simulink model "wipers_subsytem"  (R2018a)
settings: Solver=VariableStepAuto  StartTime=0.0  StopTime=inf  RelTol=1e-3
settings Model: DataTypeOverride=Double  MinMaxOverflowLogging=ForceOff  Creator=99003196  LastModifiedBy=99003188
settings DataIOCC: ReturnWorkspaceOutputs=on
settings SFSimCC: SimUseLocalCustomCode=on
settings RTWCC: RTWUseLocalCustomCode=on

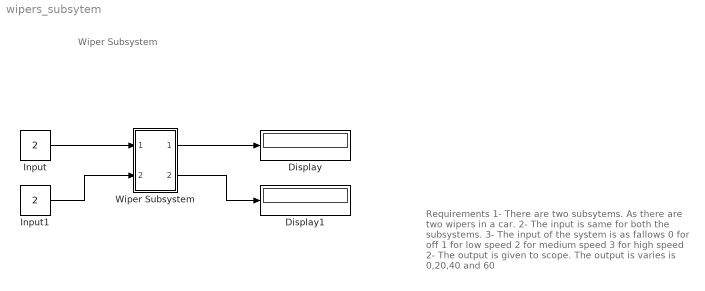
== system wipers_subsytem ==
  note: Wiper Subsystem
  note: Requirements
      | 1- There are two subsytems. As
      | there are two wipers in a car.
      | 2- The input is same for both
      | the subsystems.
      | 3- The input of the system is as fallows
      | 0 for off
      | 1 for low speed
      | 2 for medium speed
      | 3 for high speed
      | 2- The output is given to scope. The output is
      | varies is 0,20,40 and 60
  Display : Display
  Display1 : Display
  Input : Constant  Value=2
  Input1 : Constant  Value=2
  Wiper Subsystem : Subsystem
  wires:
  Input/1 -> Wiper Subsystem/1(In1)
  Wiper Subsystem/1(Out1) -> Display/1
  Input1/1 -> Wiper Subsystem/2(In2)
  Wiper Subsystem/2(Out2) -> Display1/1

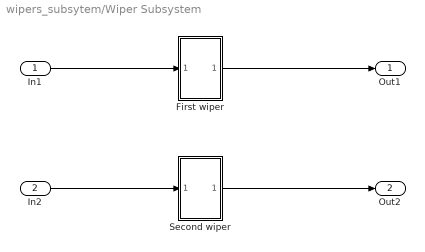
== system wipers_subsytem/Wiper Subsystem ==
  In1 : Inport
  In2 : Inport  Port=2
  First wiper : Subsystem
  Second wiper : Subsystem
  Out1 : Outport
  Out2 : Outport  Port=2
  wires:
  In1/1 -> First wiper/1(In1)
  First wiper/1(Out1) -> Out1/1
  Second wiper/1(Out1) -> Out2/1
  In2/1 -> Second wiper/1(In1)

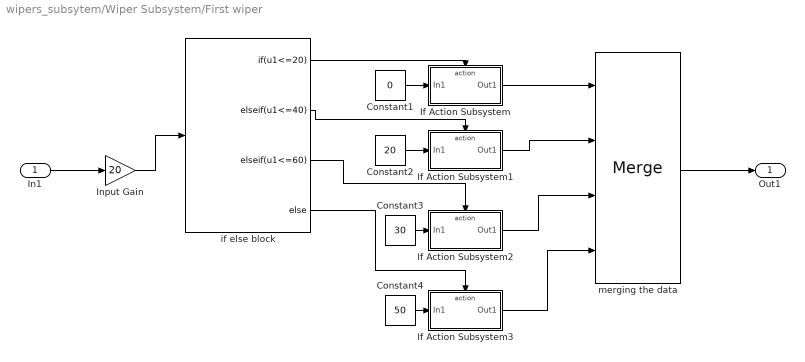
== system wipers_subsytem/Wiper Subsystem/First wiper ==
  In1 : Inport
  Constant1 : Constant  Value=0
  Constant2 : Constant  Value=20
  Constant3 : Constant  Value=30
  Constant4 : Constant  Value=50
  If Action Subsystem : Subsystem  TreatAsAtomicUnit=on
  If Action Subsystem1 : Subsystem  TreatAsAtomicUnit=on
  If Action Subsystem2 : Subsystem  TreatAsAtomicUnit=on
  If Action Subsystem3 : Subsystem  TreatAsAtomicUnit=on
  Input Gain : Gain  Gain=20
  if else block : If  IfExpression=u1<=20  ElseIfExpressions=u1<=40,u1<=60
  "merging the data " : Merge  Inputs=4
  Out1 : Outport
  wires:
  if else block/2 -> If Action Subsystem1/Action
  If Action Subsystem3/1(Out1) -> "merging the data "/4
  if else block/1 -> If Action Subsystem/Action
  if else block/3 -> If Action Subsystem2/Action
  Constant4/1 -> If Action Subsystem3/1(In1)
  If Action Subsystem/1(Out1) -> "merging the data "/1
  Constant3/1 -> If Action Subsystem2/1(In1)
  If Action Subsystem1/1(Out1) -> "merging the data "/2
  Input Gain/1 -> if else block/1
  If Action Subsystem2/1(Out1) -> "merging the data "/3
  "merging the data "/1 -> Out1/1
  In1/1 -> Input Gain/1
  Constant2/1 -> If Action Subsystem1/1(In1)
  Constant1/1 -> If Action Subsystem/1(In1)
  if else block/4 -> If Action Subsystem3/Action

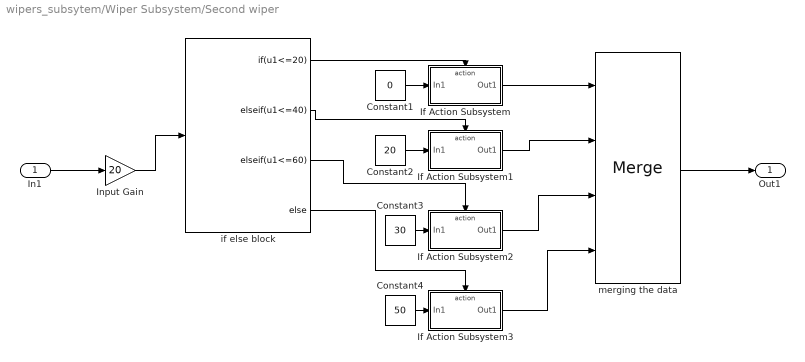
== system wipers_subsytem/Wiper Subsystem/Second wiper ==
  In1 : Inport
  Constant1 : Constant  Value=0
  Constant2 : Constant  Value=20
  Constant3 : Constant  Value=30
  Constant4 : Constant  Value=50
  If Action Subsystem : Subsystem  TreatAsAtomicUnit=on
  If Action Subsystem1 : Subsystem  TreatAsAtomicUnit=on
  If Action Subsystem2 : Subsystem  TreatAsAtomicUnit=on
  If Action Subsystem3 : Subsystem  TreatAsAtomicUnit=on
  Input Gain : Gain  Gain=20
  if else block : If  IfExpression=u1<=20  ElseIfExpressions=u1<=40,u1<=60
  "merging the data " : Merge  Inputs=4
  Out1 : Outport
  wires:
  if else block/2 -> If Action Subsystem1/Action
  If Action Subsystem3/1(Out1) -> "merging the data "/4
  if else block/1 -> If Action Subsystem/Action
  if else block/3 -> If Action Subsystem2/Action
  Constant4/1 -> If Action Subsystem3/1(In1)
  If Action Subsystem/1(Out1) -> "merging the data "/1
  Constant3/1 -> If Action Subsystem2/1(In1)
  If Action Subsystem1/1(Out1) -> "merging the data "/2
  Input Gain/1 -> if else block/1
  If Action Subsystem2/1(Out1) -> "merging the data "/3
  "merging the data "/1 -> Out1/1
  In1/1 -> Input Gain/1
  Constant2/1 -> If Action Subsystem1/1(In1)
  Constant1/1 -> If Action Subsystem/1(In1)
  if else block/4 -> If Action Subsystem3/Action

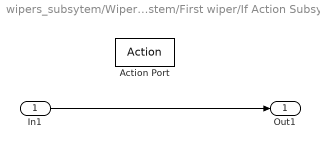
== system wipers_subsytem/Wiper Subsystem/First wiper/If Action Subsystem ==
  In1 : Inport
  Action Port : ActionPort
  Out1 : Outport
  wires:
  In1/1 -> Out1/1

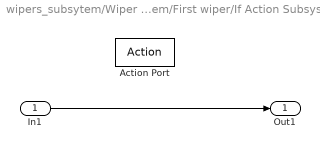
== system wipers_subsytem/Wiper Subsystem/First wiper/If Action Subsystem1 ==
  In1 : Inport
  Action Port : ActionPort
  Out1 : Outport
  wires:
  In1/1 -> Out1/1

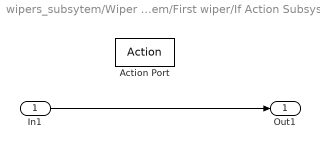
== system wipers_subsytem/Wiper Subsystem/First wiper/If Action Subsystem2 ==
  In1 : Inport
  Action Port : ActionPort
  Out1 : Outport
  wires:
  In1/1 -> Out1/1

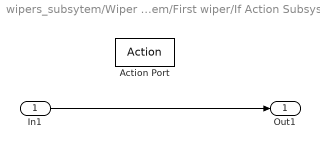
== system wipers_subsytem/Wiper Subsystem/First wiper/If Action Subsystem3 ==
  In1 : Inport
  Action Port : ActionPort
  Out1 : Outport
  wires:
  In1/1 -> Out1/1

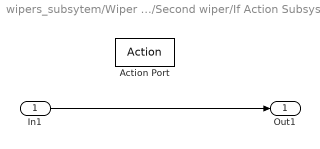
== system wipers_subsytem/Wiper Subsystem/Second wiper/If Action Subsystem ==
  In1 : Inport
  Action Port : ActionPort
  Out1 : Outport
  wires:
  In1/1 -> Out1/1

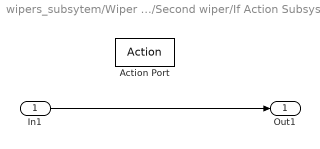
== system wipers_subsytem/Wiper Subsystem/Second wiper/If Action Subsystem1 ==
  In1 : Inport
  Action Port : ActionPort
  Out1 : Outport
  wires:
  In1/1 -> Out1/1

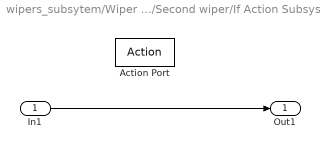
== system wipers_subsytem/Wiper Subsystem/Second wiper/If Action Subsystem2 ==
  In1 : Inport
  Action Port : ActionPort
  Out1 : Outport
  wires:
  In1/1 -> Out1/1

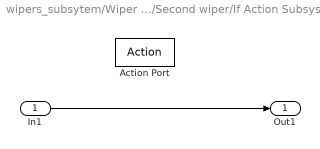
== system wipers_subsytem/Wiper Subsystem/Second wiper/If Action Subsystem3 ==
  In1 : Inport
  Action Port : ActionPort
  Out1 : Outport
  wires:
  In1/1 -> Out1/1
